simulink model "RT_Sim_Corr"  (R2020a)
settings: Solver=ode4  StartTime=0.0  StopTime=inf  FixedStep=0.004  MaxStep=TS  RelTol=1e-3
InitFcn:
  | Real_Time_Simulation_Script;
  | 
  | lego_drive_selfbalance_InitData.mdl = get_param(bdroot,'Name');
  | lego_drive_selfbalance_InitData.cs = getActiveConfigSet(lego_drive_selfbalance_InitData.mdl);
undefined symbols (not defined in the file): a_b, a_d, a_gc, a_gd, BATTERY, pwm_gain, sigbuilder_block, time_start, ts1
libraries: legoev3lib x6, simulink x4, simulink_need_slupdate x1
PreSaveFcn:
  | set_param(gcs, 'Location',[35 56 895 605])
CloseFcn:
  | clear lego_drive_selfbalance_InitData
settings Model: SimulationMode=external  ExtModeTrigDuration=2  Creator=The MathWorks Inc.  LastModifiedBy=lega
settings SolverCC: PositivePriorityOrder=on
settings DataIOCC: LimitDataPoints=on  MaxDataPoints=10000000  SaveFormat=Array  ReturnWorkspaceOutputs=off
settings OptimizationCC: ExpressionDepthLimit=2147483647  LifeSpan=Inf  MaxStackSize=64  EfficientTunableParamExpr=on
settings DebuggingCC: AlgebraicLoopMsg=none  UnderspecifiedInitializationDetection=Classic  MergeDetectMultiDrivingBlocksExec=none  Int32ToFloatConvMsg=none  ParameterPrecisionLossMsg=none  FcnCallInpInsideContextMsg=warning  StateNameClashWarn=warning  SFUnexpectedBacktrackingDiag=warning  SFNoUnconditionalDefaultTransitionDiag=warning  ArithmeticOperatorsInVariantConditions=warning
settings HardwareCC: ProdBitPerPointer=32  ProdBitPerSizeT=32  ProdBitPerPtrDiffT=32  ProdLargestAtomicInteger=Long  ProdWordSize=32  ProdHWDeviceType=ARM Compatible->ARM 9
settings ModelReferenceCC: ModelReferenceMinAlgLoopOccurrences=on  PropagateSignalLabelsOutOfModel=off
settings SFSimCC: SimUseLocalCustomCode=off  SimParseCustomCode=off  MATLABDynamicMemAlloc=off  CustomCodeUndefinedFunction=UseInterfaceOnly
settings RTWCC: SystemTargetFile=ert.tlc  HardwareBoard=LEGO MINDSTORMS EV3  TLCOptions=-aInlineSetEventsForThisBaseRateFcn=TLC_FALSE -aSuppressMultiTaskScheduler=TLC_FALSE -aRateBasedStepFcn=0  TemplateMakefile=ert_default_tmf  GenerateReport=on  RTWVerbose=off  RTWUseLocalCustomCode=off  Toolchain=Sourcery G++ Lite v2009q3  BuildConfiguration=Faster Runs  IncludeHyperlinkInReport=on  LaunchReport=on  GenerateTraceInfo=on  GenerateTraceReport=on  GenerateTraceReportSl=on  GenerateTraceReportSf=on  GenerateTraceReportEml=on
settings CodeAppCC: ForceParamTrailComments=on  IgnoreCustomStorageClasses=off  OperatorAnnotations=on  SimulinkDataObjDesc=on  SFDataObjDesc=on  MATLABFcnDesc=on  MangleLength=10  CustomSymbolStrType=$N$R$M  InsertBlockDesc=on  StateflowObjectComments=on  MATLABSourceComments=on  InternalIdentifier=Classic
settings ERTTargetCC: MultiwordLength=2048  SupportContinuousTime=on  SupportVariableSizeSignals=on  ExtMode=on  ExtModeMexArgs='10.105.0.70' 0 17725
settings ConfigComp: CovMetricSettings=dw  CovHtmlReporting=on  CovSaveCumulativeToWorkspaceVar=on  CovSaveSingleToWorkspaceVar=on  CovExternalEMLEnable=off  CovSFcnEnable=off

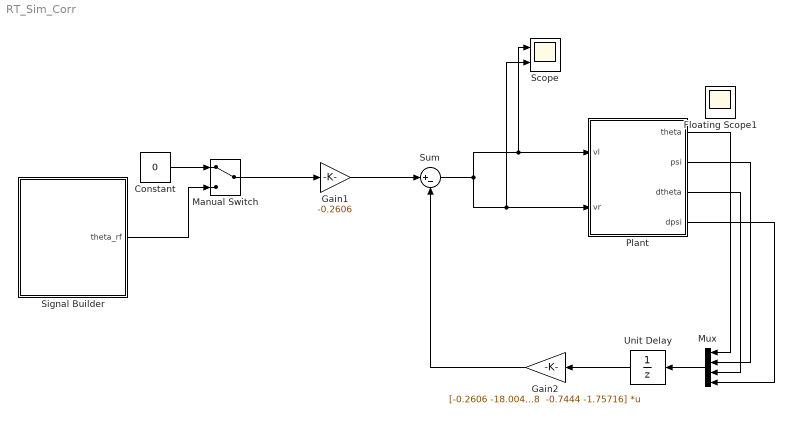
== system RT_Sim_Corr ==
  Constant : Constant  Value=0
  Gain1 : Gain  Gain=-0.2606
  Gain2 : Gain  Gain="[-0.2606 -18.0048  -0.7444 -1.75716]"  Multiplication=Matrix(K*u)
  Manual Switch : ManualSwitch
  Mux : Mux
  Plant : Subsystem
  Scope : Scope  NumInputPorts=2
  Signal Builder : Subsystem  Tag=STV Subsys  LoadFcn=sigbuilder_block('load');  StartFcn=sigbuilder_block('start');  StopFcn=sigbuilder_block('stop');  ClipboardFcn=sigbuilder_block('clipboard');  mask(Sigbuilder block){tuvar=[0:10]}
      mask help: Sigbuilder GUI
      mask init:
      | if ~strcmp(get_param(bdroot(gcbh),'SimulationStatus'),'stopped') tuvar = sigbuilder_block('maskInit'); end
      settings: CopyFcn=sigbuilder_block('copy');  DeleteFcn=sigbuilder_block('delete');  ModelCloseFcn=sigbuilder_block('modelClose');  PreSaveFcn=sigbuilder_block('preSave');  PauseFcn=sigbuilder_block('pause')  ContinueFcn=sigbuilder_block('continue')  NameChangeFcn=sigbuilder_block('namechange');  OpenFcn=sigbuilder_block('open',[146.25 169.5 569.25 349.5 ]);  CloseFcn=sigbuilder_block('close');
      mask Display: plot(0, 0, 100, 100,[2, 2, 32, 32, 2], [68, 8, 8, 68, 68],[32, 2], [38, 38], [32, 19, 2],[53, 60, 44], [32, 17, 17, 2],[16, 16, 31, 31]);txt = getActiveGroup(gcbh);text(2, 100, txt,'verticalAlignment', 'top');
  Sum : Sum  Inputs=|+-
  Unit Delay : UnitDelay  InitialCondition=[0; 0; 0; 0]  SampleTime=-1  HasFrameUpgradeWarning=on
  Floating Scope1 : Scope
  wires:
  Constant/1 -> Manual Switch/1
  Signal Builder/1(theta_rf) -> Manual Switch/2
  Plant/1(theta) -> Mux/1
  Plant/2(psi) -> Mux/2
  Plant/3(dtheta) -> Mux/3
  Plant/4(dpsi) -> Mux/4
  Manual Switch/1 -> Gain1/1
  Gain1/1 -> Sum/1
  Gain2/1 -> Sum/2
  Sum/1 -> Scope/1, Plant/1(vl), Plant/2(vr), Scope/2
  Mux/1 -> Unit Delay/1
  Unit Delay/1 -> Gain2/1

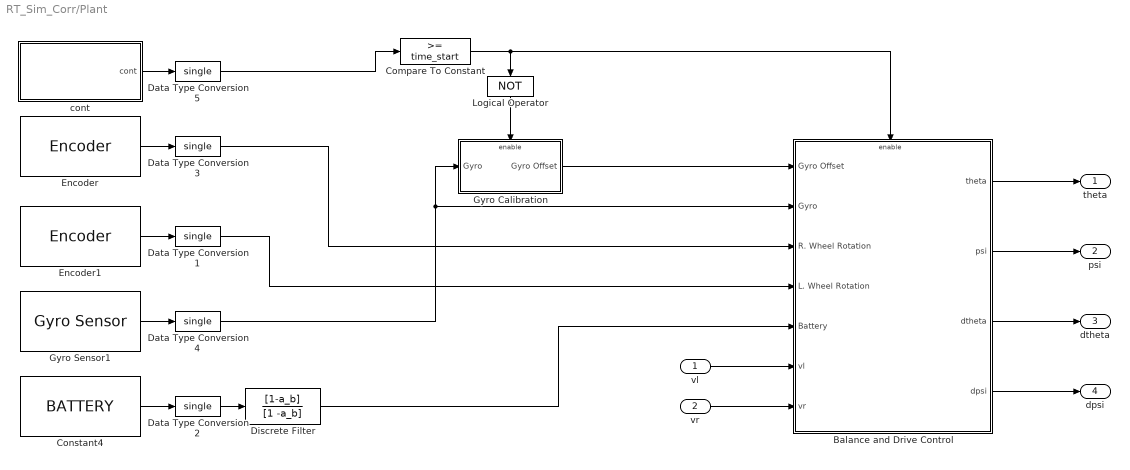
== system RT_Sim_Corr/Plant ==
  vl : Inport
  vr : Inport  Port=2
  Balance and Drive Control : Subsystem
  Compare To Constant : simulink/Logic and Bit Operations/Compare To Constant  relop=>=  const=time_start  OutDataTypeStr=boolean
  Constant4 : Constant  Value=BATTERY  OutDataTypeStr=single
  Data Type Conversion{1..5} (5 alike) : DataTypeConversion  OutDataTypeStr=single  RndMeth=Simplest
  Discrete Filter : DiscreteFilter  Numerator=[1-a_b]  Denominator=[1 -a_b]
  Encoder : legoev3lib/Encoder  portNumber=B  opMode=No reset  sampleTime=ts1
      settings: SourceProductBaseCode=LEGOEV3
  Encoder1 : legoev3lib/Encoder  portNumber=C  opMode=No reset  sampleTime=ts1
      settings: SourceProductBaseCode=LEGOEV3
  Gyro Calibration : Subsystem  TreatAsAtomicUnit=on
  Gyro Sensor1 : legoev3lib/Gyro Sensor  portNumber=4  sampleTime=ts1
      settings: SourceProductBaseCode=LEGOEV3
  Logical Operator : Logic  Operator=NOT  AllPortsSameDT=off  OutDataTypeStr=boolean
  cont : Subsystem
  theta : Outport
  psi : Outport  Port=2
  dtheta : Outport  Port=3
  dpsi : Outport  Port=4
  wires:
  Gyro Calibration/1(Gyro Offset) -> Balance and Drive Control/1(Gyro Offset)
  Data Type Conversion1/1 -> Balance and Drive Control/4(L. Wheel Rotation)
  Balance and Drive Control/3(dtheta) -> dtheta/1
  vl/1 -> Balance and Drive Control/6(vl)
  Balance and Drive Control/4(dpsi) -> dpsi/1
  Data Type Conversion3/1 -> Balance and Drive Control/3(R. Wheel Rotation)
  cont/1(cont) -> Data Type Conversion5/1
  Balance and Drive Control/1(theta) -> theta/1
  Balance and Drive Control/2(psi) -> psi/1
  Data Type Conversion4/1 -> Gyro Calibration/1(Gyro), Balance and Drive Control/2(Gyro)
  Logical Operator/1 -> Gyro Calibration/Enable
  Compare To Constant/1 -> Logical Operator/1, Balance and Drive Control/Enable
  Encoder1/1 -> Data Type Conversion1/1
  Gyro Sensor1/1 -> Data Type Conversion4/1
  Data Type Conversion2/1 -> Discrete Filter/1
  Encoder/1 -> Data Type Conversion3/1
  Constant4/1 -> Data Type Conversion2/1
  Discrete Filter/1 -> Balance and Drive Control/5(Battery)
  vr/1 -> Balance and Drive Control/7(vr)
  Data Type Conversion5/1 -> Compare To Constant/1

== system RT_Sim_Corr/Signal Builder ==
  Demux : Demux  Tag=STV Demux  Outputs=1
      settings: DisplayOption=none
  FromWs : FromWorkspace  Tag=STV FromWs  VariableName=tuvar
      SigBuilderData=|
      | common.afterFinalStr = 'Extrapolate'
      | common.sampleTime = 0
      | dataSet(1).timeRange = [0 25]
      | dataSet(1).name = 'Stand'
      | dataSet(2).timeRange = [0 25]
      | dataSet(2).name = 'Forward & Back'
      | dataSet(3).timeRange = [0 25]
      | dataSet(3).name = 'Turn'
      | dataSet(4).timeRange = [0 200]
      | dataSet(4).name = 'Approach Wall'
      | sbobj.Groups(1).Name = 'Stand'
      | sbobj.Groups(1).Signals.Name = 'theta_rf'
      | sbobj.Groups(1).Signals.XData = [0 25]
      | sbobj.Groups(1).Signals.YData = [0 0]
      | sbobj.Groups(1).TimeRange = [0 25]
      | sbobj.Groups(2).Name = 'Forward & Back'
      | sbobj.Groups(2).Signals.Name = 'theta_rf'
      | sbobj.Groups(2).Signals.XData = [0 5 5 8.5 8.5 15 15 20 20 25]
      | sbobj.Groups(2).Signals.YData = [0 0 0.48 0.48 0 0 -0.5 -0.5 0 0]
      | sbobj.Groups(2).TimeRange = [0 25]
      | sbobj.Groups(3).Name = 'Turn'
      | sbobj.Groups(3).Signals.Name = 'theta_rf'
      | sbobj.Groups(3).Signals.XData = [0 10 10 15 15 20 20 25]
      | sbobj.Groups(3).Signals.YData = [0 0 0.5 0.5 0 0 0.49 0.49]
      | sbobj.Groups(3).TimeRange = [0 25]
      | sbobj.Groups(4).Name = 'Approach Wall'
      | sbobj.Groups(4).Signals.Name = 'theta_rf'
      | sbobj.Groups(4).Signals.XData = [0 10 12 140 188.5 200]
      | sbobj.Groups(4).Signals.YData = [0 0 0 84 84 84]
      | sbobj.Groups(4).TimeRange = [0 200]
  theta_rf : Outport  Tag=STV Outport
  wires:
  FromWs/1 -> Demux/1
  Demux/1 -> theta_rf/1

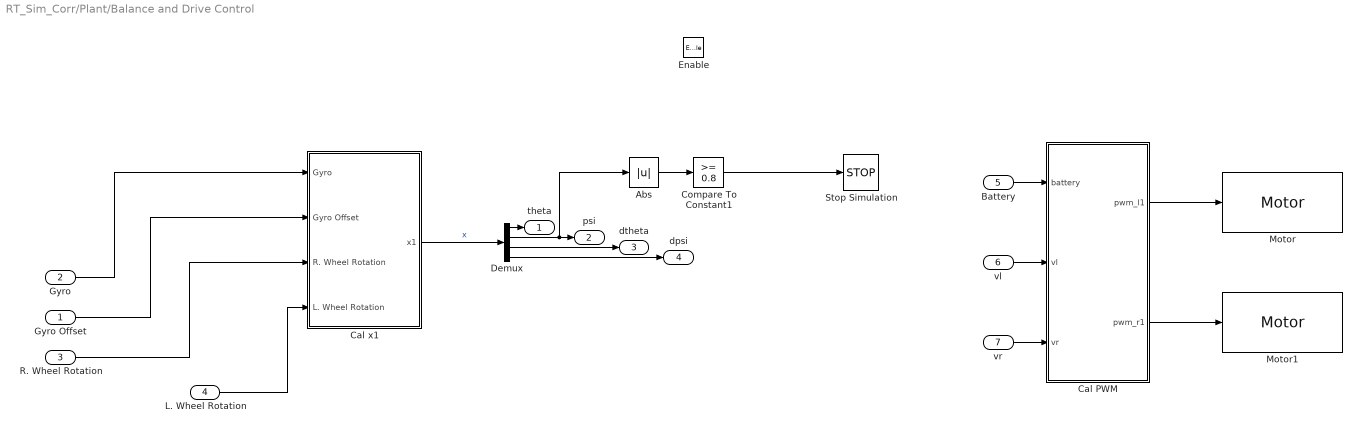
== system RT_Sim_Corr/Plant/Balance and Drive Control ==
  Gyro Offset : Inport
  Gyro : Inport  Port=2
  R. Wheel Rotation : Inport  Port=3
  L. Wheel Rotation : Inport  Port=4
  Battery : Inport  Port=5
  vl : Inport  Port=6
  vr : Inport  Port=7
  Enable : EnablePort
  Abs : Abs
  Cal PWM : Subsystem
  Cal x1 : Subsystem
  Compare To Constant1 : simulink/Logic and Bit Operations/Compare To Constant  relop=>=  const=0.8  OutDataTypeStr=boolean
  Demux : Demux
  Motor : legoev3lib/Motor  sportNumber=B  sstopAction=Brake
  Motor1 : legoev3lib/Motor  sportNumber=C  sstopAction=Brake
  Stop Simulation : Stop
  theta : Outport
  psi : Outport  Port=2
  dtheta : Outport  Port=3
  dpsi : Outport  Port=4
  wires:
  L. Wheel Rotation/1 -> Cal x1/4(L. Wheel Rotation)
  R. Wheel Rotation/1 -> Cal x1/3(R. Wheel Rotation)
  Gyro/1 -> Cal x1/1(Gyro)
  Gyro Offset/1 -> Cal x1/2(Gyro Offset)
  Compare To Constant1/1 -> Stop Simulation/1
  Abs/1 -> Compare To Constant1/1
  Battery/1 -> Cal PWM/1(battery)
  Cal PWM/1(pwm_l1) -> Motor/1
  Cal PWM/2(pwm_r1) -> Motor1/1
  Cal x1/1(x1) -> Demux/1  "x"
  Demux/1 -> theta/1
  Demux/2 -> Abs/1, psi/1
  Demux/3 -> dtheta/1
  Demux/4 -> dpsi/1
  vl/1 -> Cal PWM/2(vl)
  vr/1 -> Cal PWM/3(vr)

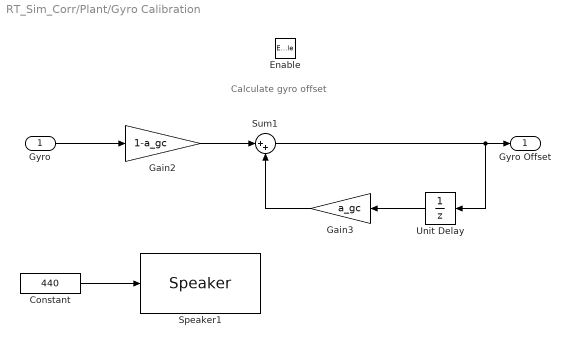
== system RT_Sim_Corr/Plant/Gyro Calibration ==
  note: Calculate gyro offset
  Gyro : Inport
  Enable : EnablePort
  Constant : Constant  Value=440  OutDataTypeStr=uint32  SampleTime=0.2
  Gain2 : Gain  Gain=1-a_gc  OutDataTypeStr=Inherit: Same as input  ParamDataTypeStr=Inherit: Same as input
  Gain3 : Gain  Gain=a_gc  OutDataTypeStr=Inherit: Same as input  ParamDataTypeStr=Inherit: Same as input
  Speaker1 : legoev3lib/Speaker  sinputMode=Frequency only  sspeakerFreq=100  sspeakerVolume=25  sspeakerDuration=100
      settings: SourceProductBaseCode=LEGOEV3
  Sum1 : Sum  Inputs=|++  OutDataTypeStr=Inherit: Same as first input
  Unit Delay : UnitDelay  SampleTime=-1  HasFrameUpgradeWarning=on
  Gyro Offset : Outport
  wires:
  Gain3/1 -> Sum1/2
  Unit Delay/1 -> Gain3/1
  Sum1/1 -> Unit Delay/1, Gyro Offset/1
  Gain2/1 -> Sum1/1
  Gyro/1 -> Gain2/1
  Constant/1 -> Speaker1/1

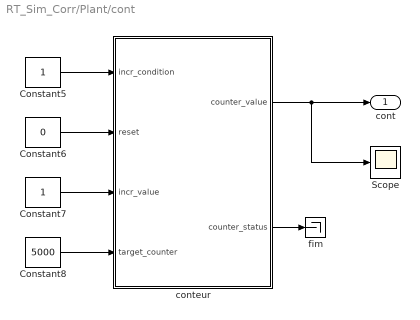
== system RT_Sim_Corr/Plant/cont ==
  Constant5 : Constant  OutDataTypeStr=single  SampleTime=ts1
  Constant6 : Constant  Value=0  OutDataTypeStr=single  SampleTime=ts1
  Constant7 : Constant  OutDataTypeStr=single  SampleTime=ts1
  Constant8 : Constant  Value=5000  OutDataTypeStr=single
  Scope : Scope
  conteur : Subsystem
  fim : Terminator
  cont : Outport
  wires:
  conteur/2(counter_status) -> fim/1
  Constant8/1 -> conteur/4(target_counter)
  conteur/1(counter_value) -> Scope/1, cont/1
  Constant7/1 -> conteur/3(incr_value)
  Constant5/1 -> conteur/1(incr_condition)
  Constant6/1 -> conteur/2(reset)

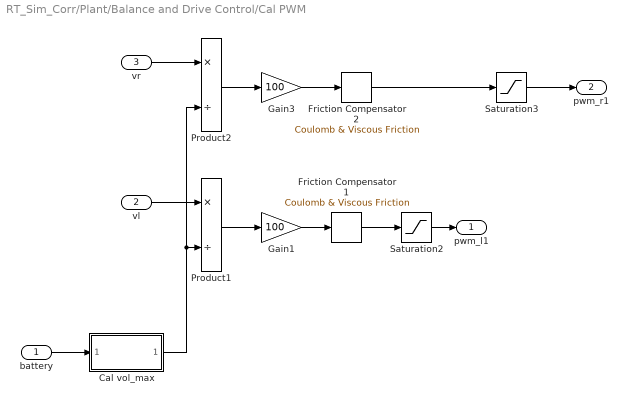
== system RT_Sim_Corr/Plant/Balance and Drive Control/Cal PWM ==
  battery : Inport
  vl : Inport  Port=2
  vr : Inport  Port=3
  Cal vol_max : Subsystem
  Friction Compensator1 : simulink/Discontinuities/Coulomb & Viscous Friction  offset=pwm_offset  gain=pwm_gain
      settings: AttributesFormatString=gain = %<gain>\noffset = %<offset>
  Friction Compensator2 : simulink/Discontinuities/Coulomb & Viscous Friction  offset=pwm_offset  gain=pwm_gain
      settings: AttributesFormatString=gain = %<gain>\noffset = %<offset>
  Gain1 : Gain  Gain=100  OutDataTypeStr=Inherit: Same as input  ParamDataTypeStr=Inherit: Same as input
  Gain3 : Gain  Gain=100  OutDataTypeStr=Inherit: Same as input  ParamDataTypeStr=Inherit: Same as input
  Product1 : Product  Inputs=*/  RndMeth=Simplest  OutDataTypeStr=Inherit: Same as first input
  Product2 : Product  Inputs=*/  RndMeth=Simplest  OutDataTypeStr=Inherit: Same as first input
  Saturation2 : Saturate  UpperLimit=100  LowerLimit=-100
      settings: AttributesFormatString=max = %<UpperLimit>\nmin = %<LowerLimit>
  Saturation3 : Saturate  UpperLimit=100  LowerLimit=-100
      settings: AttributesFormatString=max = %<UpperLimit>\nmin = %<LowerLimit>
  pwm_l1 : Outport
  pwm_r1 : Outport  Port=2
  wires:
  Product1/1 -> Gain1/1
  Saturation2/1 -> pwm_l1/1
  Product2/1 -> Gain3/1
  Cal vol_max/1(vol_max) -> Product2/2, Product1/2
  Gain1/1 -> Friction Compensator1/1
  vr/1 -> Product2/1
  vl/1 -> Product1/1
  Gain3/1 -> Friction Compensator2/1
  battery/1 -> Cal vol_max/1(battery)
  Saturation3/1 -> pwm_r1/1
  Friction Compensator1/1 -> Saturation2/1
  Friction Compensator2/1 -> Saturation3/1

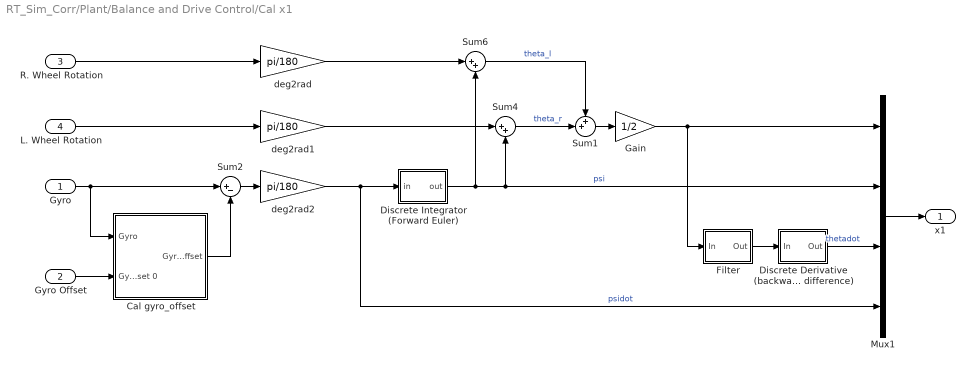
== system RT_Sim_Corr/Plant/Balance and Drive Control/Cal x1 ==
  Gyro : Inport
  Gyro Offset : Inport  Port=2
  R. Wheel Rotation : Inport  Port=3
  L. Wheel Rotation : Inport  Port=4
  Cal gyro_offset : Subsystem
  Discrete Derivative (backward difference) : Subsystem
  Discrete Integrator (Forward Euler) : Subsystem
  Filter : Subsystem
  Gain : Gain  Gain=1/2  OutDataTypeStr=Inherit: Same as input  ParamDataTypeStr=Inherit: Same as input
  Mux1 : Mux
  Sum1 : Sum  Inputs=++|  OutDataTypeStr=Inherit: Same as first input
  Sum2 : Sum  Inputs=|+-  OutDataTypeStr=Inherit: Same as first input
  Sum4 : Sum  Inputs=|++  OutDataTypeStr=Inherit: Same as first input
  Sum6 : Sum  Inputs=|++  OutDataTypeStr=Inherit: Same as first input
  deg2rad : Gain  Gain=pi/180  OutDataTypeStr=Inherit: Same as input  ParamDataTypeStr=Inherit: Same as input
  deg2rad1 : Gain  Gain=pi/180  OutDataTypeStr=Inherit: Same as input  ParamDataTypeStr=Inherit: Same as input
  deg2rad2 : Gain  Gain=pi/180  OutDataTypeStr=Inherit: Same as input  ParamDataTypeStr=Inherit: Same as input
  x1 : Outport
  wires:
  Gain/1 -> Mux1/1, Filter/1(In)
  Filter/1(Out) -> Discrete Derivative (backward difference)/1(In)
  deg2rad2/1 -> Mux1/4, Discrete Integrator (Forward Euler)/1(in)  "psidot"
  Sum1/1 -> Gain/1
  Sum4/1 -> Sum1/2  "theta_r"
  Sum6/1 -> Sum1/1  "theta_l"
  Discrete Derivative (backward difference)/1(Out) -> Mux1/3  "thetadot"
  L. Wheel Rotation/1 -> deg2rad1/1
  R. Wheel Rotation/1 -> deg2rad/1
  deg2rad/1 -> Sum6/1
  Mux1/1 -> x1/1
  deg2rad1/1 -> Sum4/1
  Gyro/1 -> Sum2/1, Cal gyro_offset/1(Gyro)
  Sum2/1 -> deg2rad2/1
  Cal gyro_offset/1(Gyro Offset) -> Sum2/2
  Gyro Offset/1 -> Cal gyro_offset/2(Gyro Offset 0)
  Discrete Integrator (Forward Euler)/1(out) -> Sum6/2, Mux1/2, Sum4/2  "psi"

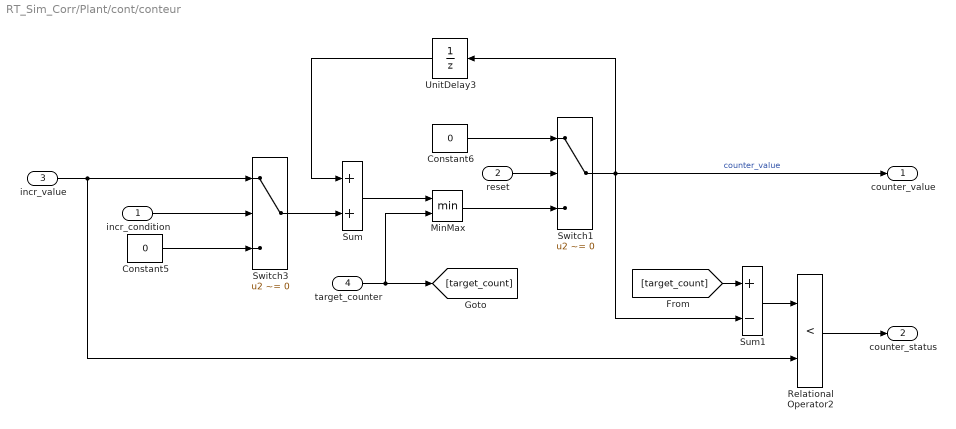
== system RT_Sim_Corr/Plant/cont/conteur ==
  incr_condition : Inport
  reset : Inport  Port=2
  incr_value : Inport  Port=3
  target_counter : Inport  Port=4
  Constant5 : Constant  Value=0  OutDataTypeStr=Inherit: Inherit via back propagation
  Constant6 : Constant  Value=0  OutDataTypeStr=Inherit: Inherit via back propagation
  MinMax : MinMax  Inputs=2
  Relational Operator2 : RelationalOperator  Operator=<  OutDataTypeStr=boolean  RndMeth=Nearest
  Sum : Sum
  Sum1 : Sum  Inputs=+-
  Switch1 : Switch  Criteria=u2 ~= 0  InputSameDT=on
  Switch3 : Switch  Criteria=u2 ~= 0  InputSameDT=on
  UnitDelay3 : UnitDelay  SampleTime=-1  HasFrameUpgradeWarning=on
      settings: AttributesFormatString=|
      | Initial = %<X0>
      | tsample = %<SampleTime>
  counter_value : Outport
  counter_status : Outport  Port=2
  wires:
  Switch3/1 -> Sum/2
  [target_count] -> Sum1/1
  Sum/1 -> MinMax/1
  Relational Operator2/1 -> counter_status/1
  reset/1 -> Switch1/2
  MinMax/1 -> Switch1/3
  target_counter/1 -> [target_count], MinMax/2
  Sum1/1 -> Relational Operator2/1
  incr_value/1 -> Switch3/1, Relational Operator2/2
  Constant6/1 -> Switch1/1
  Switch1/1 -> counter_value/1, Sum1/2, UnitDelay3/1  "counter_value"
  UnitDelay3/1 -> Sum/1
  Constant5/1 -> Switch3/3
  incr_condition/1 -> Switch3/2

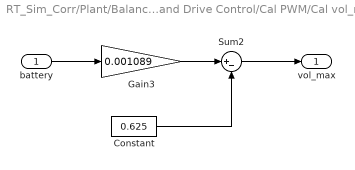
== system RT_Sim_Corr/Plant/Balance and Drive Control/Cal PWM/Cal vol_max ==
  battery : Inport
  Constant : Constant  Value=0.625  OutDataTypeStr=single  SampleTime=-1
      settings: AttributesFormatString=DataType = %<OutDataTypeStr>
  Gain3 : Gain  Gain=0.001089  OutDataTypeStr=Inherit: Same as input  ParamDataTypeStr=Inherit: Same as input
  Sum2 : Sum  Inputs=|+-  OutDataTypeStr=Inherit: Same as first input
  vol_max : Outport
  wires:
  Constant/1 -> Sum2/2
  Sum2/1 -> vol_max/1
  Gain3/1 -> Sum2/1
  battery/1 -> Gain3/1

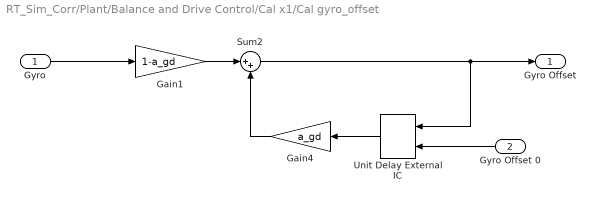
== system RT_Sim_Corr/Plant/Balance and Drive Control/Cal x1/Cal gyro_offset ==
  Gyro : Inport
  Gyro Offset 0 : Inport  Port=2
  Gain1 : Gain  Gain=1-a_gd  OutDataTypeStr=Inherit: Same as input  ParamDataTypeStr=Inherit: Same as input
  Gain4 : Gain  Gain=a_gd  OutDataTypeStr=Inherit: Same as input  ParamDataTypeStr=Inherit: Same as input
  Sum2 : Sum  Inputs=|++  OutDataTypeStr=Inherit: Same as first input
  Unit Delay External IC : simulink_need_slupdate/Unit Delay External IC  tsamp=-1
      settings: SourceProductBaseCode=SL
  Gyro Offset : Outport
  wires:
  Gyro/1 -> Gain1/1
  Gyro Offset 0/1 -> Unit Delay External IC/2
  Gain1/1 -> Sum2/1
  Sum2/1 -> Gyro Offset/1, Unit Delay External IC/1
  Unit Delay External IC/1 -> Gain4/1
  Gain4/1 -> Sum2/2

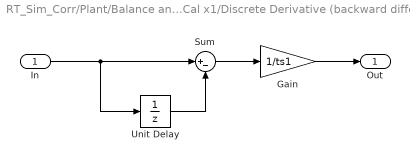
== system RT_Sim_Corr/Plant/Balance and Drive Control/Cal x1/Discrete Derivative (backward difference) ==
  In : Inport
  Gain : Gain  Gain=1/ts1  OutDataTypeStr=Inherit: Same as input  ParamDataTypeStr=Inherit: Same as input
  Sum : Sum  Inputs=|+-  OutDataTypeStr=Inherit: Same as first input
  Unit Delay : UnitDelay  SampleTime=-1  HasFrameUpgradeWarning=on
  Out : Outport
  wires:
  Gain/1 -> Out/1
  In/1 -> Sum/1, Unit Delay/1
  Unit Delay/1 -> Sum/2
  Sum/1 -> Gain/1

== system RT_Sim_Corr/Plant/Balance and Drive Control/Cal x1/Discrete Integrator (Forward Euler) ==
  in : Inport
  Gain : Gain  Gain=ts1  OutDataTypeStr=Inherit: Same as input  ParamDataTypeStr=Inherit: Same as input
  Sum : Sum  Inputs=|++  OutDataTypeStr=Inherit: Same as first input
  Unit Delay : UnitDelay  SampleTime=-1  HasFrameUpgradeWarning=on
  out : Outport
  wires:
  Unit Delay/1 -> Sum/2, out/1
  Gain/1 -> Sum/1
  Sum/1 -> Unit Delay/1
  in/1 -> Gain/1

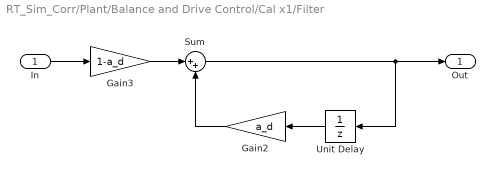
== system RT_Sim_Corr/Plant/Balance and Drive Control/Cal x1/Filter ==
  In : Inport
  Gain2 : Gain  Gain=a_d  OutDataTypeStr=Inherit: Same as input  ParamDataTypeStr=Inherit: Same as input
  Gain3 : Gain  Gain=1-a_d  OutDataTypeStr=Inherit: Same as input  ParamDataTypeStr=Inherit: Same as input
  Sum : Sum  Inputs=|++  OutDataTypeStr=Inherit: Same as first input
  Unit Delay : UnitDelay  SampleTime=-1  HasFrameUpgradeWarning=on
  Out : Outport
  wires:
  In/1 -> Gain3/1
  Gain3/1 -> Sum/1
  Gain2/1 -> Sum/2
  Unit Delay/1 -> Gain2/1
  Sum/1 -> Out/1, Unit Delay/1
